simulink model "acm_sil"  (R2024b)
settings: Solver=VariableStepAuto  StartTime=0.0  StopTime=2  RelTol=1e-3
libraries: peripheral_utilities x2, spsAsynchronousMachineSIUnitsLib x1, spsControlledVoltageSourceLib x1, gmp_sil_core_pack x1, sps_lib x1
settings Model: Creator=javnson  LastModifiedBy=javnson

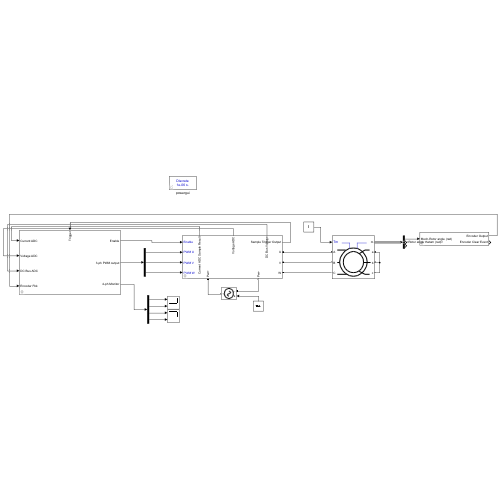
[thumbnail: Simulink's stored preview of the top-level diagram]
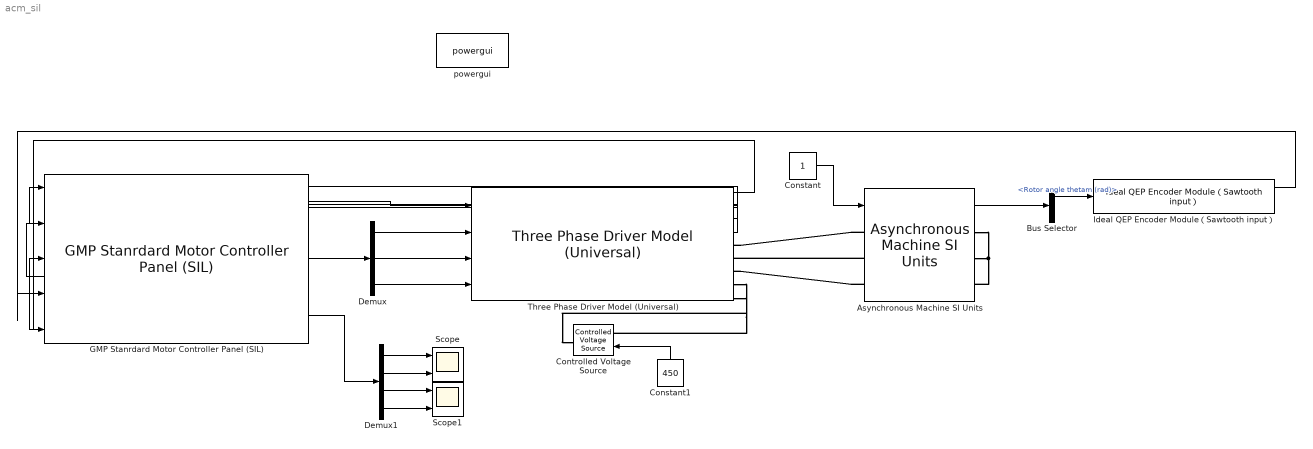
== system acm_sil ==
  Asynchronous Machine SI Units : spsAsynchronousMachineSIUnitsLib/Asynchronous Machine SI Units  RotorType=Wound  PresetModel=No  MechanicalLoad=Torque Tm  ShowDetailedParameters=on  ReferenceFrame=Rotor  Units=SI  MeasurementBus=off  NominalParameters=[1.845e+04 400 50]  VoltageRatio=1  Stator=[0.5968 0.0003495]  Rotor=[0.6258 0.005473]  Cage1=[0.4155 0.002066]  Cage2=[0.4168 0.0003495]  Lm=0.0354  Mechanical=[0.05 0.005879 2]  PolePairs=2  InitialConditions=[0 0 0 0 0 0 0 0]  SimulateSaturation=off  Saturation=[14.03593122, 27.81365428, 53.79336849, 72.68890987, 97.98006896, 148.6815601, 215.7428561, 302.9841135, 428.7778367 ; 230, 322, 414, 460, 506, 552, 598, 644, 690]  LoadFlowParameters=1492000  TsPowergui=0  TsBlock=-1  IterativeModel=Trapezoidal non iterative  IterativeDiscreteModel=Trapezoidal non iterative  Pmec=1.492e+006
  Bus Selector : BusSelector  OutputSignals="Mechanical.Rotor angle thetam (rad),Rotor measurements.Rotor current  iq (A),Rotor measurements.Rotor current  id (A)"
  Constant : Constant
  Constant1 : Constant  Value=450
  Controlled Voltage Source : spsControlledVoltageSourceLib/Controlled Voltage Source  Initialize=on  Source_Type=AC  Amplitude=0  Phase=0  Frequency=0  Measurements=None
  Demux : Demux  Outputs=3
  Demux1 : Demux
  GMP Stanrdard Motor Controller Panel (SIL) : gmp_sil_core_pack/GMP Stanrdard Motor Controller Panel (SIL)
      settings: SourceProductName=GMP SIL Core Utilities
  Ideal QEP Encoder Module（Sawtooth input） : peripheral_utilities/Ideal QEP Encoder Module（Sawtooth input）  QEP_LINE=2000
      settings: SourceProductName=Virtual Peripheral Utilities
  Scope : Scope  NumInputPorts=2
  Scope1 : Scope  NumInputPorts=2
  Three Phase Driver Model (Universal) : peripheral_utilities/Three Phase Driver Model (Universal)  fswitch=10e3  CMP_MAX=10000  Deadband_Upper=75  Deadband_Lower=75  Deadband_us=0.75  phase_shift=0  R_mosfet_on=0.1  Lon=0  Rd=0.01  Vf=0.3  Rs=1e5  Cs=inf  Rsap=0.005  ADC_GAIN=20  ADC_BIT=12  ADC_REFERENCE=3.3  ADC_BIAS=1.65  ADC_INIT=0  VOLTAGE_ADC_GAIN=0.04049127  VOLTAGE_ADC_BIT=12  VOLTAGE_ADC_REFERENCE=3.3  VOLTAGE_ADC_VOLTAGE=0  VOLTAGE_ADC_INIT=0  VOLTAGE_ADC_CUT_FREQ=1143.4  DCBUS_ADC_GAIN=0.04049127  DCBUS_ADC_BIT=12  DCBUS_ADC_REFERENCE=3.3  DCBUS_ADC_BIAS=0  DCBUS_ADC_INIT=0
      settings: SourceProductName=Virtual Peripheral Utilities
  powergui : sps_lib/powergui  Priority=1  SimulationMode=Discrete  SampleTime=1e-6  frequency=60  Iterations=50  frequencyindice=50  Pbase=100e6  ErrMax=1e-4  UnitsV=kV  UnitsW=MW  buscounter=0  FunctionMessages=off  echomessages=off  EnableUseOfTLC=off  CurrentSourceSwitches=off  DisableSnubberDevices=off  DisableRonSwitches=off  DisableVfSwitches=off  DisplayEquations=off  AutomaticDiscreteSolvers=off  SolverType=Tustin/Backward Euler (TBE)  Interpol=off  ExternalGateDelay=off  methode=off  Ts=100  x0status=blocks  SPID=on  SwTol=0  HookPort=off  NonlinearTolerance=1e-4  nMaxIteration=100  ContinueOnMaxIteration=off  RestoreLinks=warning  ResistiveCurrentMeasurement=off  Frange=[0:2:500]  Ylog=off  Xlog=on  ShowGrid=off  save=off  variable=ZData  structure=0  ZoomFFT=off  StartTime=0.0  cycles=1  DisplayStyle=1  fundamental=60  FreqAxis=off  MaxFrequency=1000  frequencyindicesteady=1  RmsSteady=1  display=off
  wires:
  Constant/1 -> Asynchronous Machine SI Units/1
  Constant1/1 -> Controlled Voltage Source/1
  Demux/1 -> Three Phase Driver Model (Universal)/2
  Demux/2 -> Three Phase Driver Model (Universal)/3
  Demux/3 -> Three Phase Driver Model (Universal)/4
  GMP Stanrdard Motor Controller Panel (SIL)/2 -> Demux/1
  GMP Stanrdard Motor Controller Panel (SIL)/1 -> Three Phase Driver Model (Universal)/1
  GMP Stanrdard Motor Controller Panel (SIL)/3 -> Demux1/1
  Demux1/1 -> Scope/1
  Demux1/2 -> Scope/2
  Demux1/3 -> Scope1/1
  Demux1/4 -> Scope1/2
  Three Phase Driver Model (Universal)/1 -> GMP Stanrdard Motor Controller Panel (SIL)/5
  Three Phase Driver Model (Universal)/2 -> GMP Stanrdard Motor Controller Panel (SIL)/1
  Three Phase Driver Model (Universal)/3 -> GMP Stanrdard Motor Controller Panel (SIL)/2
  Three Phase Driver Model (Universal)/4 -> GMP Stanrdard Motor Controller Panel (SIL)/3
  Asynchronous Machine SI Units/1 -> Bus Selector/1
  Bus Selector/1 -> Ideal QEP Encoder Module（Sawtooth input）/1  "<Rotor angle thetam (rad)>"
  Ideal QEP Encoder Module（Sawtooth input）/1 -> GMP Stanrdard Motor Controller Panel (SIL)/4
  connections:
  Asynchronous Machine SI Units/LConn1 -- Three Phase Driver Model (Universal)/RConn1
  Asynchronous Machine SI Units/LConn2 -- Three Phase Driver Model (Universal)/RConn2
  Asynchronous Machine SI Units/LConn3 -- Three Phase Driver Model (Universal)/RConn3
  Asynchronous Machine SI Units/RConn1 -- Asynchronous Machine SI Units/RConn2 -- Asynchronous Machine SI Units/RConn3
  Three Phase Driver Model (Universal)/RConn5 -- Controlled Voltage Source/LConn1
  Three Phase Driver Model (Universal)/RConn4 -- Controlled Voltage Source/RConn1
